simulink model "controller"  (R2023b)
settings: Solver=FixedStepAuto  StartTime=0.0  StopTime=100  FixedStep=1/100  RelTol=1e-3
undefined symbols (not defined in the file): MAX_TORQUE, MAX_TORQUE_REVERSE
settings Model: Creator=DAUIN-Win10  LastModifiedBy=RSKALA
settings OptimizationCC: ReuseModelBlockBuffer=off
settings DebuggingCC: UnconnectedInputMsg=warning  UnconnectedOutputMsg=warning  UnconnectedLineMsg=warning
settings ModelReferenceCC: EnableRefExpFcnMdlSchedulingChecks=on
settings RTWCC: DLArmComputeVersion=19.05

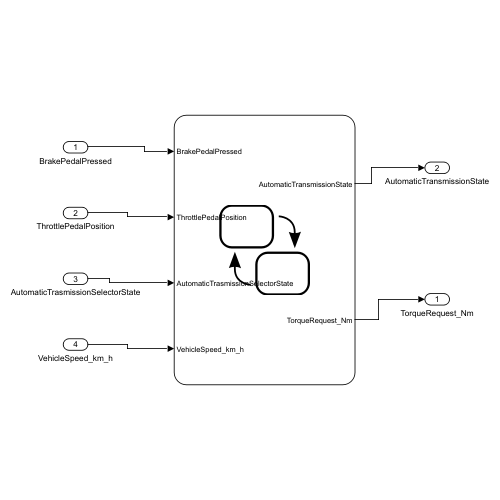
[thumbnail: Simulink's stored preview of the top-level diagram]
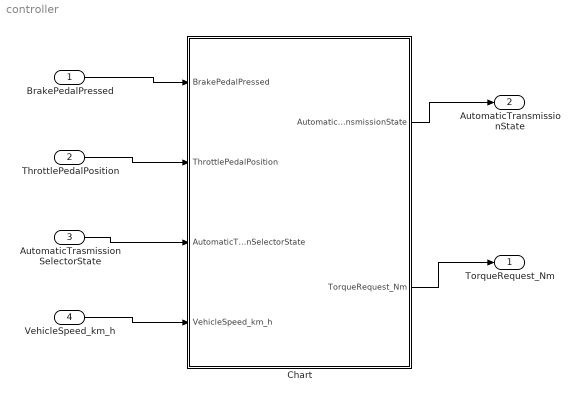
== system controller ==
  BrakePedalPressed : Inport  OutDataTypeStr=boolean
  ThrottlePedalPosition : Inport  Port=2  OutDataTypeStr=single
  AutomaticTrasmissionSelectorState : Inport  Port=3  OutDataTypeStr=Enum: TransmissionState
  VehicleSpeed_km_h : Inport  Port=4  OutDataTypeStr=single  Unit=km/h
  Chart : Stateflow chart  TreatAsAtomicUnit=on
  TorqueRequest_Nm : Outport  OutDataTypeStr=single  Unit=N*m
  AutomaticTransmissionState : Outport  Port=2  OutDataTypeStr=Enum: TransmissionState
  wires:
  BrakePedalPressed/1 -> Chart/1(BrakePedalPressed)
  ThrottlePedalPosition/1 -> Chart/2(ThrottlePedalPosition)
  AutomaticTrasmissionSelectorState/1 -> Chart/3(AutomaticTrasmissionSelectorState)
  VehicleSpeed_km_h/1 -> Chart/4(VehicleSpeed_km_h)
  Chart/1(AutomaticTransmissionState) -> AutomaticTransmissionState/1
  Chart/2(TorqueRequest_Nm) -> TorqueRequest_Nm/1

== stateflow chart controller/Chart ==
  state P
    en:
    AutomaticTransmissionState=TransmissionState.Park;
    du:
    TorqueRequest_Nm=0;
  state B
    en:
    AutomaticTransmissionState=TransmissionState.Brake;
    state Accelerate
      du:
      TorqueRequest_Nm=MAX_TORQUE*(3/2)*(ThrottlePedalPosition-(1/3));
    state Stop
      en:
      TorqueRequest_Nm=0;
    state Decelerate
      du:
      TorqueRequest_Nm=-MAX_TORQUE*(1-3*ThrottlePedalPosition);
    (default) -> Accelerate
    Stop -> Accelerate : [ThrottlePedalPosition>=1/3]
    Accelerate -> Decelerate : [ThrottlePedalPosition<=(1/3)]
    Decelerate -> Accelerate [order 2] : [ThrottlePedalPosition>(1/3)]
    Decelerate -> Stop [order 1] : [VehicleSpeed_km_h<=0]
  state N
    en:
    AutomaticTransmissionState=TransmissionState.Neutral;
    du:
    TorqueRequest_Nm=0;
  state R
    en:
    AutomaticTransmissionState=TransmissionState.Reverse;
    du:
    TorqueRequest_Nm=ThrottlePedalPosition*-MAX_TORQUE_REVERSE;
  state D
    en:
    AutomaticTransmissionState=TransmissionState.Drive;
    du:
    TorqueRequest_Nm=ThrottlePedalPosition*MAX_TORQUE;
  (default) -> P
  P -> N : [AutomaticTrasmissionSelectorState~=TransmissionState.Park&BrakePedalPressed==1]
  N -> P [order 1] : [AutomaticTrasmissionSelectorState==TransmissionState.Park&BrakePedalPressed==1&abs(VehicleSpeed_km_h)<5]
  N -> D [order 2] : [AutomaticTrasmissionSelectorState==TransmissionState.Drive||AutomaticTrasmissionSelectorState==TransmissionState.Brake&BrakePedalPressed==1&VehicleSpeed_km_h>-5]
  R -> N : [AutomaticTrasmissionSelectorState~=TransmissionState.Reverse]
  D -> N [order 2] : [AutomaticTrasmissionSelectorState==TransmissionState.Neutral || AutomaticTrasmissionSelectorState==TransmissionState.Reverse || AutomaticTrasmissionSelectorState==TransmissionState.Park]
  D -> B [order 1] : [ ThrottlePedalPosition>(1/3)&AutomaticTrasmissionSelectorState==TransmissionState.Brake]
  N -> R [order 3] : [AutomaticTrasmissionSelectorState==TransmissionState.Reverse&BrakePedalPressed==1&VehicleSpeed_km_h<5]
  B -> D : [AutomaticTrasmissionSelectorState~=TransmissionState.Brake]
  data: BrakePedalPressed input boolean; ThrottlePedalPosition input single; AutomaticTrasmissionSelectorState input Enum: TransmissionState; VehicleSpeed_km_h input single; AutomaticTransmissionState output Enum: TransmissionState; TorqueRequest_Nm output single; MAX_TORQUE_REVERSE parameter; MAX_TORQUE parameter
